simulink model "DiagCCaller_TestHarness"  (R2019a)
settings: Solver=FixedStepDiscrete  StartTime=0.0  StopTime=10.0  FixedStep=0.1  RelTol=1e-3  EnableMultiTasking=on
undefined symbols (not defined in the file): Dem_EventStatusType, sigbuilder_block
(part 1 of 4)
settings Model: Creator=E9911830  LastModifiedBy=E9911830
settings SolverCC: AutoInsertRateTranBlk=on
settings DataIOCC: ReturnWorkspaceOutputs=off
settings OptimizationCC: DefaultParameterBehavior=Inlined  EnhancedBackFolding=on  PassReuseOutputArgsAs=Individual arguments  ZeroExternalMemoryAtStartup=off  ZeroInternalMemoryAtStartup=off  OptimizeBlockOrder=speed  DifferentSizesBufferReuse=on  OptimizationCustomize=off
settings DebuggingCC: ParameterTunabilityLossMsg=error
settings SFSimCC: SimCustomHeaderCode="#include \"DiagDebounce.h\""  SimUserSources=DiagDebounce.c  MATLABDynamicMemAlloc=off
settings RTWCC: SystemTargetFile=ert.tlc  GenCodeOnly=on  TemplateMakefile=ert_default_tmf  GenerateReport=on  IncludeHyperlinkInReport=on  LaunchReport=on  GenerateTraceInfo=on  GenerateTraceReport=on  GenerateTraceReportSl=on  GenerateTraceReportSf=on  GenerateTraceReportEml=on
settings CodeAppCC: ForceParamTrailComments=on  IgnoreCustomStorageClasses=off  OperatorAnnotations=on  SimulinkDataObjDesc=on  SFDataObjDesc=on  InsertBlockDesc=on
settings ERTTargetCC: TargetLangStandard=C99 (ISO)  GenerateSampleERTMain=on  InlinedParameterPlacement=NonHierarchical  ERTCustomFileTemplate=example_file_process.tlc

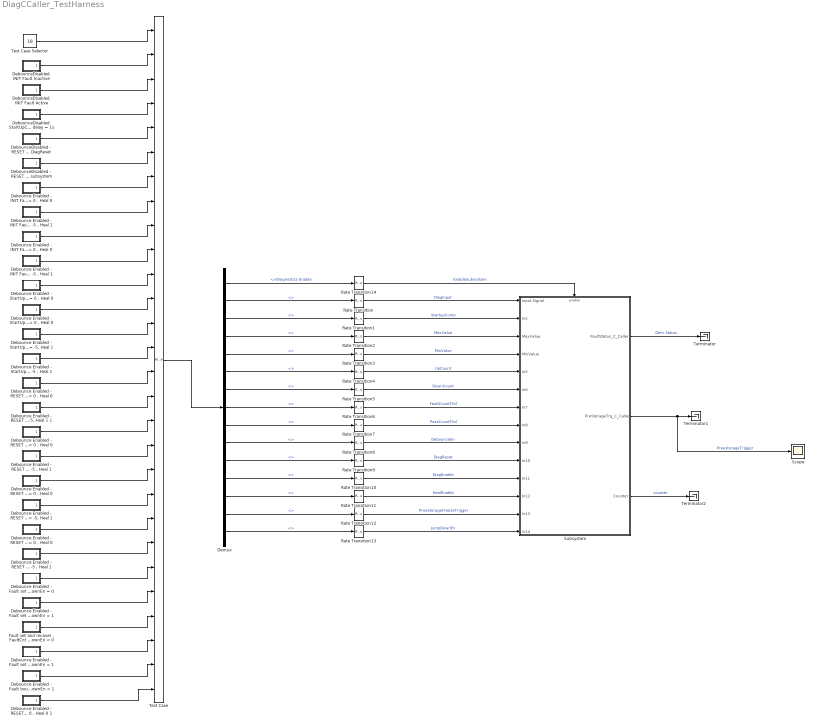
== system DiagCCaller_TestHarness ==
  "Debounce Enabled - Fault bounces , FaultCnt = 10, PassCnt = -5 , Heal =1, JumpDownEn = 1 " : Subsystem
  "Debounce Enabled - Fault set and recover , FaultCnt = 10, PassCnt = -5 , Heal =1, JumpDownEn = 1 " : Subsystem
  "Debounce Enabled - Fault set and recover , FaultCnt = 10, PassCnt = 0 , Heal =0, JumpDownEn = 0 " : Subsystem
  "Debounce Enabled - Fault set and recover , FaultCnt = 10, PassCnt = 0 , Heal =0, JumpDownEn = 1 " : Subsystem
  "Debounce Enabled - INIT Fault Active , FaultCnt = 10, PassCnt = -5 , Heal 1 " : Subsystem
  "Debounce Enabled - INIT Fault Active , FaultCnt = 10, PassCnt = 0 , Heal 0 " : Subsystem
  "Debounce Enabled - INIT Fault Inactive , FaultCnt = 10, PassCnt = -5 , Heal 1 " : Subsystem
  "Debounce Enabled - INIT Fault Inactive , FaultCnt = 10, PassCnt = 0 , Heal 0 " : Subsystem
  "Debounce Enabled - RESET by Calibration ,Fault Active, FaultCnt = 10, PassCnt = -5, Heal 1 1" : Subsystem
  "Debounce Enabled - RESET by Calibration ,Fault Active, FaultCnt = 10, PassCnt = 0 , Heal 0 " : Subsystem
  "Debounce Enabled - RESET by Calibration ,Fault Inactive , FaultCnt = 10, PassCnt = 0 , Heal 0 " : Subsystem
  "Debounce Enabled - RESET by Calibration ,Fault Inactive,  FaultCnt = 10, PassCnt = -5 , Heal 1 " : Subsystem
  "Debounce Enabled - RESET by Disable\\Enable subsystem,Fault Active, FaultCnt = 10, PassCnt = -5, Heal 1 " : Subsystem
  "Debounce Enabled - RESET by Disable\\Enable subsystem,Fault Active, FaultCnt = 10, PassCnt = 0 , Heal 0 " : Subsystem
  "Debounce Enabled - RESET by Disable\\Enable subsystem,Fault Inactive,  FaultCnt = 10, PassCnt = -5 , Heal 1 " : Subsystem
  "Debounce Enabled - RESET by Disable\\Enable subsystem,Fault Inactive, , FaultCnt = 10, PassCnt = 0 , Heal 0 " : Subsystem
  "Debounce Enabled - RESET by Disable\\Enable subsystem,Fault Inactive, , FaultCnt = 10, PassCnt = 0 , Heal 0 1" : Subsystem
  "Debounce Enabled - StartUpComp delay = 1s, Fault Active , FaultCnt = 10, PassCnt = -5 , Heal 1 " : Subsystem
  "Debounce Enabled - StartUpComp delay = 1s, Fault Active , FaultCnt = 10, PassCnt = 0 , Heal 0 " : Subsystem
  "Debounce Enabled - StartUpComp delay = 1s, Fault Inactive , FaultCnt = 10, PassCnt = -5, Heal 1 " : Subsystem
  "Debounce Enabled - StartUpComp delay = 1s, Fault Inactive , FaultCnt = 10, PassCnt = 0 , Heal 0 " : Subsystem
  "DebounceDisabled - RESET by Calibration DiagReset " : Subsystem
  "DebounceDisabled - RESET by Disable\\Enable subsystem " : Subsystem
  "DebounceDisabled INIT Fault Active " : Subsystem
  "DebounceDisabled INIT Fault Inactive " : Subsystem
  "DebounceDisabled StartUpComp delay = 1s " : Subsystem
  Demux : Demux  Outputs=15
  "Fault set and recover , FaultCnt = 10, PassCnt = -5 , Heal =1, JumpDownEn = 0 " : Subsystem
  Rate Transition{,1..14} (15 alike) : RateTransition  OutPortSampleTime=.1
  Scope : Scope
  Subsystem : Subsystem
  Terminator : Terminator
  Terminator1 : Terminator
  Terminator2 : Terminator
  Test Case : MultiPortSwitch  Inputs=27
  Test Case Selector : Constant  Value=18
  wires:
  Rate Transition/1 -> Subsystem/1(Input Signal)  "DiagInput"
  Demux/2 -> Rate Transition/1  "<>"
  Demux/3 -> Rate Transition1/1  "<>"
  Demux/4 -> Rate Transition2/1  "<>"
  Demux/5 -> Rate Transition3/1  "<>"
  Demux/6 -> Rate Transition4/1  "<>"
  Demux/7 -> Rate Transition5/1  "<>"
  Demux/8 -> Rate Transition6/1  "<>"
  Demux/9 -> Rate Transition7/1  "<>"
  Demux/10 -> Rate Transition8/1  "<>"
  Demux/11 -> Rate Transition9/1  "<>"
  Demux/12 -> Rate Transition10/1  "<>"
  Demux/13 -> Rate Transition11/1  "<>"
  Demux/14 -> Rate Transition12/1  "<>"
  Demux/15 -> Rate Transition13/1  "<>"
  Subsystem/1(FaultStatus_C_Caller) -> Terminator/1  "Dem Status"
  Subsystem/2(PreStorageTrg_C_Caller) -> Scope/1, Terminator1/1  "PreestorageTrigger"
  Demux/1 -> Rate Transition14/1  "<>Diagnostics Enable"
  "DebounceDisabled INIT Fault Inactive "/1(Out1) -> Test Case/2
  Test Case/1 -> Demux/1
  Test Case Selector/1 -> Test Case/1
  "DebounceDisabled INIT Fault Active "/1(Out1) -> Test Case/3
  "DebounceDisabled StartUpComp delay = 1s "/1(Out1) -> Test Case/4
  Rate Transition1/1 -> Subsystem/2(In2)  "StartupComp"
  Rate Transition4/1 -> Subsystem/5(In5)  "UpCount"
  Rate Transition5/1 -> Subsystem/6(In6)  "DownCount"
  Rate Transition6/1 -> Subsystem/7(In7)  "FaultCountThd"
  Rate Transition7/1 -> Subsystem/8(In8)  "PassCountThd"
  Rate Transition8/1 -> Subsystem/9(In9)  "DebounceEn"
  Rate Transition9/1 -> Subsystem/10(In10)  "DiagReset"
  Rate Transition10/1 -> Subsystem/11(In11)  "DiagEnable"
  Rate Transition11/1 -> Subsystem/12(In12)  "HealEnable"
  Rate Transition12/1 -> Subsystem/13(In13)  "PreestorageFreezeTrigger"
  Rate Transition13/1 -> Subsystem/14(In14)  "JumpDownEn"
  Rate Transition14/1 -> Subsystem/Enable  "EnableSubsystem"
  "DebounceDisabled - RESET by Calibration DiagReset "/1(Out1) -> Test Case/5
  Subsystem/3(Counter) -> Terminator2/1  "counter"
  "DebounceDisabled - RESET by Disable\\Enable subsystem "/1(Out1) -> Test Case/6
  "Debounce Enabled - INIT Fault Inactive , FaultCnt = 10, PassCnt = 0 , Heal 0 "/1(Out1) -> Test Case/7
  "Debounce Enabled - INIT Fault Inactive , FaultCnt = 10, PassCnt = -5 , Heal 1 "/1(Out1) -> Test Case/8
  "Debounce Enabled - INIT Fault Active , FaultCnt = 10, PassCnt = 0 , Heal 0 "/1(Out1) -> Test Case/9
  "Debounce Enabled - INIT Fault Active , FaultCnt = 10, PassCnt = -5 , Heal 1 "/1(Out1) -> Test Case/10
  "Debounce Enabled - StartUpComp delay = 1s, Fault Inactive , FaultCnt = 10, PassCnt = 0 , Heal 0 "/1(Out1) -> Test Case/11
  "Debounce Enabled - StartUpComp delay = 1s, Fault Active , FaultCnt = 10, PassCnt = 0 , Heal 0 "/1(Out1) -> Test Case/12
  "Debounce Enabled - StartUpComp delay = 1s, Fault Inactive , FaultCnt = 10, PassCnt = -5, Heal 1 "/1(Out1) -> Test Case/13
  "Debounce Enabled - StartUpComp delay = 1s, Fault Active , FaultCnt = 10, PassCnt = -5 , Heal 1 "/1(Out1) -> Test Case/14
  "Debounce Enabled - RESET by Calibration ,Fault Active, FaultCnt = 10, PassCnt = 0 , Heal 0 "/1(Out1) -> Test Case/15
  "Debounce Enabled - RESET by Calibration ,Fault Active, FaultCnt = 10, PassCnt = -5, Heal 1 1"/1(Out1) -> Test Case/16
  "Debounce Enabled - RESET by Calibration ,Fault Inactive , FaultCnt = 10, PassCnt = 0 , Heal 0 "/1(Out1) -> Test Case/17
  "Debounce Enabled - RESET by Calibration ,Fault Inactive,  FaultCnt = 10, PassCnt = -5 , Heal 1 "/1(Out1) -> Test Case/18
  "Debounce Enabled - RESET by Disable\\Enable subsystem,Fault Active, FaultCnt = 10, PassCnt = 0 , Heal 0 "/1(Out1) -> Test Case/19
  "Debounce Enabled - RESET by Disable\\Enable subsystem,Fault Active, FaultCnt = 10, PassCnt = -5, Heal 1 "/1(Out1) -> Test Case/20
  "Debounce Enabled - RESET by Disable\\Enable subsystem,Fault Inactive, , FaultCnt = 10, PassCnt = 0 , Heal 0 "/1(Out1) -> Test Case/21
  "Debounce Enabled - RESET by Disable\\Enable subsystem,Fault Inactive,  FaultCnt = 10, PassCnt = -5 , Heal 1 "/1(Out1) -> Test Case/22
  "Debounce Enabled - Fault set and recover , FaultCnt = 10, PassCnt = 0 , Heal =0, JumpDownEn = 1 "/1(Out1) -> Test Case/24
  "Debounce Enabled - Fault set and recover , FaultCnt = 10, PassCnt = 0 , Heal =0, JumpDownEn = 0 "/1(Out1) -> Test Case/23
  "Fault set and recover , FaultCnt = 10, PassCnt = -5 , Heal =1, JumpDownEn = 0 "/1(Out1) -> Test Case/25
  "Debounce Enabled - Fault set and recover , FaultCnt = 10, PassCnt = -5 , Heal =1, JumpDownEn = 1 "/1(Out1) -> Test Case/26
  "Debounce Enabled - Fault bounces , FaultCnt = 10, PassCnt = -5 , Heal =1, JumpDownEn = 1 "/1(Out1) -> Test Case/27
  Rate Transition2/1 -> Subsystem/3(MaxValue)  "MaxValue"
  Rate Transition3/1 -> Subsystem/4(MinValue)  "MinValue"
  "Debounce Enabled - RESET by Disable\\Enable subsystem,Fault Inactive, , FaultCnt = 10, PassCnt = 0 , Heal 0 1"/1(Out1) -> Test Case/28

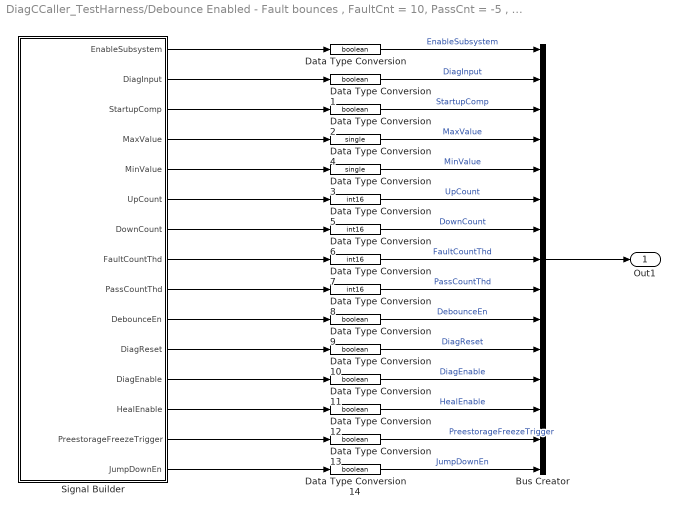
== system DiagCCaller_TestHarness/Debounce Enabled - Fault bounces , FaultCnt = 10, PassCnt = -5 , Heal =1, JumpDownEn = 1  ==
  Bus Creator : BusCreator  Inputs=15
  Data Type Conversion{,1..2,9..14} (9 alike) : DataTypeConversion  OutDataTypeStr=boolean
  Data Type Conversion3 : DataTypeConversion  OutDataTypeStr=single
  Data Type Conversion4 : DataTypeConversion  OutDataTypeStr=single
  Data Type Conversion{5..8} (4 alike) : DataTypeConversion  OutDataTypeStr=int16
  Signal Builder : Subsystem  Tag=STV Subsys  LoadFcn=sigbuilder_block('load');  StartFcn=sigbuilder_block('start');  StopFcn=sigbuilder_block('stop');  ClipboardFcn=sigbuilder_block('clipboard');  TreatAsAtomicUnit=on  mask(Sigbuilder block){tuvar=[0:10]}
      mask help: Simulink:masks:SigbuilderBlock_MD
      mask init:
      | if ~strcmp(get_param(bdroot(gcbh),'SimulationStatus'),'stopped') tuvar = sigbuilder_block('maskInit'); end
      settings: CopyFcn=sigbuilder_block('copy');  DeleteFcn=sigbuilder_block('delete');  ModelCloseFcn=sigbuilder_block('modelClose');  PreSaveFcn=sigbuilder_block('preSave');  PauseFcn=sigbuilder_block('pause');  ContinueFcn=sigbuilder_block('continue');  NameChangeFcn=sigbuilder_block('namechange');  OpenFcn=sigbuilder_block('open',[0 30 1152 561.6 ]);  CloseFcn=sigbuilder_block('close');
      mask Display: plot(0, 0, 100, 100,[2, 2, 32, 32, 2], [68, 8, 8, 68, 68],[32, 2], [38, 38], [32, 19, 2],[53, 60, 44], [32, 17, 17, 2],[16, 16, 31, 31]);txt = getActiveGroup(gcbh);text(2, 100, txt,'verticalAlignment', 'top');
  Out1 : Outport
  wires:
  Bus Creator/1 -> Out1/1
  Signal Builder/2(DiagInput) -> Data Type Conversion1/1
  Signal Builder/3(StartupComp) -> Data Type Conversion2/1
  Signal Builder/4(MaxValue) -> Data Type Conversion4/1
  Signal Builder/5(MinValue) -> Data Type Conversion3/1
  Signal Builder/6(UpCount) -> Data Type Conversion5/1
  Signal Builder/7(DownCount) -> Data Type Conversion6/1
  Signal Builder/8(FaultCountThd) -> Data Type Conversion7/1
  Signal Builder/9(PassCountThd) -> Data Type Conversion8/1
  Signal Builder/10(DebounceEn) -> Data Type Conversion9/1
  Signal Builder/11(DiagReset) -> Data Type Conversion10/1
  Signal Builder/12(DiagEnable) -> Data Type Conversion11/1
  Signal Builder/13(HealEnable) -> Data Type Conversion12/1
  Signal Builder/14(PreestorageFreezeTrigger) -> Data Type Conversion13/1
  Signal Builder/15(JumpDownEn) -> Data Type Conversion14/1
  Signal Builder/1(EnableSubsystem) -> Data Type Conversion/1
  Data Type Conversion/1 -> Bus Creator/1  "EnableSubsystem"
  Data Type Conversion1/1 -> Bus Creator/2  "DiagInput"
  Data Type Conversion2/1 -> Bus Creator/3  "StartupComp"
  Data Type Conversion4/1 -> Bus Creator/4  "MaxValue"
  Data Type Conversion3/1 -> Bus Creator/5  "MinValue"
  Data Type Conversion5/1 -> Bus Creator/6  "UpCount"
  Data Type Conversion6/1 -> Bus Creator/7  "DownCount"
  Data Type Conversion7/1 -> Bus Creator/8  "FaultCountThd"
  Data Type Conversion8/1 -> Bus Creator/9  "PassCountThd"
  Data Type Conversion9/1 -> Bus Creator/10  "DebounceEn"
  Data Type Conversion10/1 -> Bus Creator/11  "DiagReset"
  Data Type Conversion11/1 -> Bus Creator/12  "DiagEnable"
  Data Type Conversion12/1 -> Bus Creator/13  "HealEnable"
  Data Type Conversion13/1 -> Bus Creator/14  "PreestorageFreezeTrigger"
  Data Type Conversion14/1 -> Bus Creator/15  "JumpDownEn"

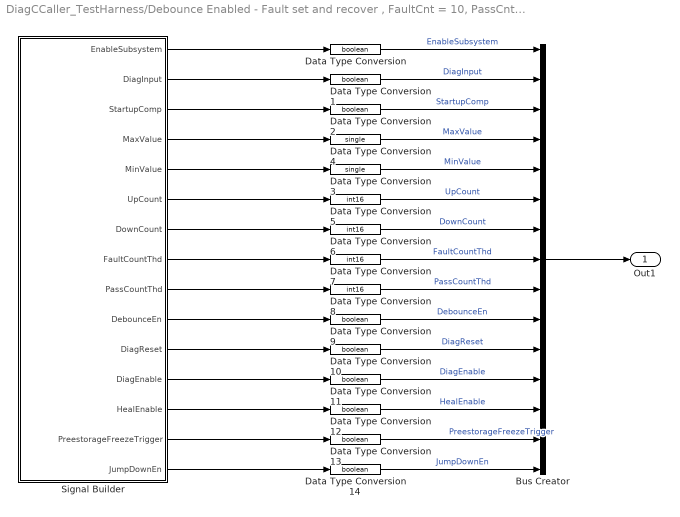
== system DiagCCaller_TestHarness/Debounce Enabled - Fault set and recover , FaultCnt = 10, PassCnt = -5 , Heal =1, JumpDownEn = 1  ==
  Bus Creator : BusCreator  Inputs=15
  Data Type Conversion{,1..2,9..14} (9 alike) : DataTypeConversion  OutDataTypeStr=boolean
  Data Type Conversion3 : DataTypeConversion  OutDataTypeStr=single
  Data Type Conversion4 : DataTypeConversion  OutDataTypeStr=single
  Data Type Conversion{5..8} (4 alike) : DataTypeConversion  OutDataTypeStr=int16
  Signal Builder : Subsystem  Tag=STV Subsys  LoadFcn=sigbuilder_block('load');  StartFcn=sigbuilder_block('start');  StopFcn=sigbuilder_block('stop');  ClipboardFcn=sigbuilder_block('clipboard');  TreatAsAtomicUnit=on  mask(Sigbuilder block){tuvar=[0:10]}
      mask help: Simulink:masks:SigbuilderBlock_MD
      mask init:
      | if ~strcmp(get_param(bdroot(gcbh),'SimulationStatus'),'stopped') tuvar = sigbuilder_block('maskInit'); end
      settings: CopyFcn=sigbuilder_block('copy');  DeleteFcn=sigbuilder_block('delete');  ModelCloseFcn=sigbuilder_block('modelClose');  PreSaveFcn=sigbuilder_block('preSave');  PauseFcn=sigbuilder_block('pause');  ContinueFcn=sigbuilder_block('continue');  NameChangeFcn=sigbuilder_block('namechange');  OpenFcn=sigbuilder_block('open',[5.4 30 1141.2 522.6 ]);  CloseFcn=sigbuilder_block('close');
      mask Display: plot(0, 0, 100, 100,[2, 2, 32, 32, 2], [68, 8, 8, 68, 68],[32, 2], [38, 38], [32, 19, 2],[53, 60, 44], [32, 17, 17, 2],[16, 16, 31, 31]);txt = getActiveGroup(gcbh);text(2, 100, txt,'verticalAlignment', 'top');
  Out1 : Outport
  wires:
  Data Type Conversion14/1 -> Bus Creator/15  "JumpDownEn"
  Data Type Conversion13/1 -> Bus Creator/14  "PreestorageFreezeTrigger"
  Data Type Conversion12/1 -> Bus Creator/13  "HealEnable"
  Data Type Conversion11/1 -> Bus Creator/12  "DiagEnable"
  Data Type Conversion10/1 -> Bus Creator/11  "DiagReset"
  Data Type Conversion9/1 -> Bus Creator/10  "DebounceEn"
  Data Type Conversion8/1 -> Bus Creator/9  "PassCountThd"
  Data Type Conversion7/1 -> Bus Creator/8  "FaultCountThd"
  Data Type Conversion6/1 -> Bus Creator/7  "DownCount"
  Data Type Conversion5/1 -> Bus Creator/6  "UpCount"
  Data Type Conversion3/1 -> Bus Creator/5  "MinValue"
  Data Type Conversion4/1 -> Bus Creator/4  "MaxValue"
  Data Type Conversion2/1 -> Bus Creator/3  "StartupComp"
  Data Type Conversion1/1 -> Bus Creator/2  "DiagInput"
  Data Type Conversion/1 -> Bus Creator/1  "EnableSubsystem"
  Signal Builder/1(EnableSubsystem) -> Data Type Conversion/1
  Signal Builder/15(JumpDownEn) -> Data Type Conversion14/1
  Signal Builder/14(PreestorageFreezeTrigger) -> Data Type Conversion13/1
  Signal Builder/13(HealEnable) -> Data Type Conversion12/1
  Signal Builder/12(DiagEnable) -> Data Type Conversion11/1
  Signal Builder/11(DiagReset) -> Data Type Conversion10/1
  Signal Builder/10(DebounceEn) -> Data Type Conversion9/1
  Signal Builder/9(PassCountThd) -> Data Type Conversion8/1
  Signal Builder/8(FaultCountThd) -> Data Type Conversion7/1
  Signal Builder/7(DownCount) -> Data Type Conversion6/1
  Signal Builder/6(UpCount) -> Data Type Conversion5/1
  Signal Builder/5(MinValue) -> Data Type Conversion3/1
  Signal Builder/4(MaxValue) -> Data Type Conversion4/1
  Signal Builder/3(StartupComp) -> Data Type Conversion2/1
  Signal Builder/2(DiagInput) -> Data Type Conversion1/1
  Bus Creator/1 -> Out1/1

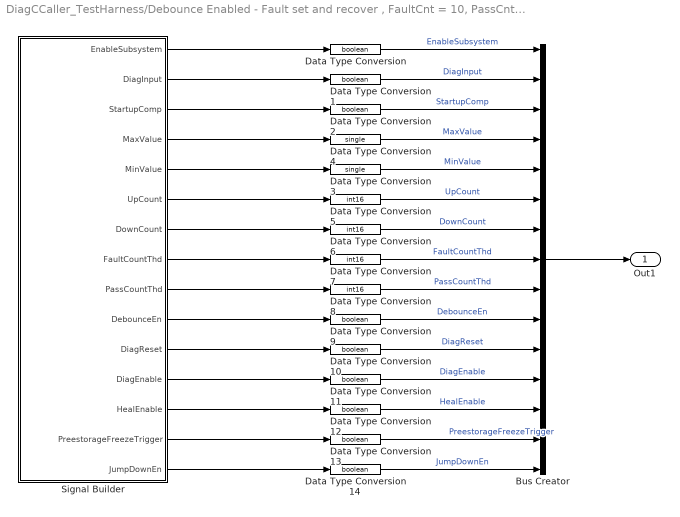
== system DiagCCaller_TestHarness/Debounce Enabled - Fault set and recover , FaultCnt = 10, PassCnt = 0 , Heal =0, JumpDownEn = 0  ==
  Bus Creator : BusCreator  Inputs=15
  Data Type Conversion{,1..2,9..14} (9 alike) : DataTypeConversion  OutDataTypeStr=boolean
  Data Type Conversion3 : DataTypeConversion  OutDataTypeStr=single
  Data Type Conversion4 : DataTypeConversion  OutDataTypeStr=single
  Data Type Conversion{5..8} (4 alike) : DataTypeConversion  OutDataTypeStr=int16
  Signal Builder : Subsystem  Tag=STV Subsys  LoadFcn=sigbuilder_block('load');  StartFcn=sigbuilder_block('start');  StopFcn=sigbuilder_block('stop');  ClipboardFcn=sigbuilder_block('clipboard');  TreatAsAtomicUnit=on  mask(Sigbuilder block){tuvar=[0:10]}
      mask help: Simulink:masks:SigbuilderBlock_MD
      mask init:
      | if ~strcmp(get_param(bdroot(gcbh),'SimulationStatus'),'stopped') tuvar = sigbuilder_block('maskInit'); end
      settings: CopyFcn=sigbuilder_block('copy');  DeleteFcn=sigbuilder_block('delete');  ModelCloseFcn=sigbuilder_block('modelClose');  PreSaveFcn=sigbuilder_block('preSave');  PauseFcn=sigbuilder_block('pause');  ContinueFcn=sigbuilder_block('continue');  NameChangeFcn=sigbuilder_block('namechange');  OpenFcn=sigbuilder_block('open',[5.4 30 1141.2 522.6 ]);  CloseFcn=sigbuilder_block('close');
      mask Display: plot(0, 0, 100, 100,[2, 2, 32, 32, 2], [68, 8, 8, 68, 68],[32, 2], [38, 38], [32, 19, 2],[53, 60, 44], [32, 17, 17, 2],[16, 16, 31, 31]);txt = getActiveGroup(gcbh);text(2, 100, txt,'verticalAlignment', 'top');
  Out1 : Outport
  wires:
  Data Type Conversion14/1 -> Bus Creator/15  "JumpDownEn"
  Data Type Conversion13/1 -> Bus Creator/14  "PreestorageFreezeTrigger"
  Data Type Conversion12/1 -> Bus Creator/13  "HealEnable"
  Data Type Conversion11/1 -> Bus Creator/12  "DiagEnable"
  Data Type Conversion10/1 -> Bus Creator/11  "DiagReset"
  Data Type Conversion9/1 -> Bus Creator/10  "DebounceEn"
  Data Type Conversion8/1 -> Bus Creator/9  "PassCountThd"
  Data Type Conversion7/1 -> Bus Creator/8  "FaultCountThd"
  Data Type Conversion6/1 -> Bus Creator/7  "DownCount"
  Data Type Conversion5/1 -> Bus Creator/6  "UpCount"
  Data Type Conversion3/1 -> Bus Creator/5  "MinValue"
  Data Type Conversion4/1 -> Bus Creator/4  "MaxValue"
  Data Type Conversion2/1 -> Bus Creator/3  "StartupComp"
  Data Type Conversion1/1 -> Bus Creator/2  "DiagInput"
  Data Type Conversion/1 -> Bus Creator/1  "EnableSubsystem"
  Signal Builder/1(EnableSubsystem) -> Data Type Conversion/1
  Signal Builder/15(JumpDownEn) -> Data Type Conversion14/1
  Signal Builder/14(PreestorageFreezeTrigger) -> Data Type Conversion13/1
  Signal Builder/13(HealEnable) -> Data Type Conversion12/1
  Signal Builder/12(DiagEnable) -> Data Type Conversion11/1
  Signal Builder/11(DiagReset) -> Data Type Conversion10/1
  Signal Builder/10(DebounceEn) -> Data Type Conversion9/1
  Signal Builder/9(PassCountThd) -> Data Type Conversion8/1
  Signal Builder/8(FaultCountThd) -> Data Type Conversion7/1
  Signal Builder/7(DownCount) -> Data Type Conversion6/1
  Signal Builder/6(UpCount) -> Data Type Conversion5/1
  Signal Builder/5(MinValue) -> Data Type Conversion3/1
  Signal Builder/4(MaxValue) -> Data Type Conversion4/1
  Signal Builder/3(StartupComp) -> Data Type Conversion2/1
  Signal Builder/2(DiagInput) -> Data Type Conversion1/1
  Bus Creator/1 -> Out1/1

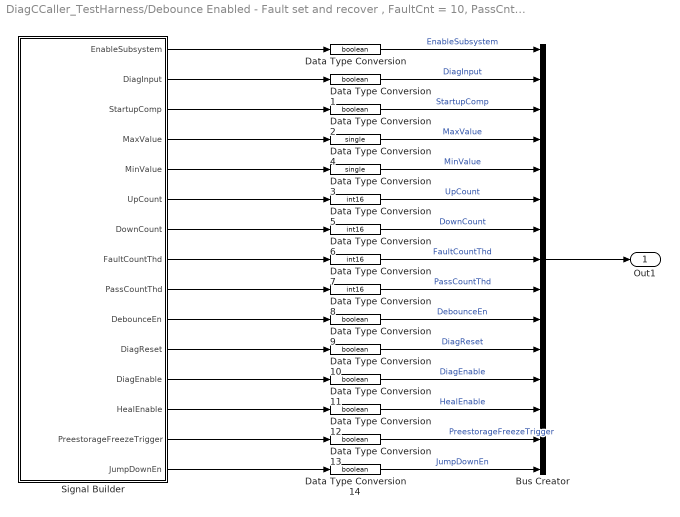
== system DiagCCaller_TestHarness/Debounce Enabled - Fault set and recover , FaultCnt = 10, PassCnt = 0 , Heal =0, JumpDownEn = 1  ==
  Bus Creator : BusCreator  Inputs=15
  Data Type Conversion{,1..2,9..14} (9 alike) : DataTypeConversion  OutDataTypeStr=boolean
  Data Type Conversion3 : DataTypeConversion  OutDataTypeStr=single
  Data Type Conversion4 : DataTypeConversion  OutDataTypeStr=single
  Data Type Conversion{5..8} (4 alike) : DataTypeConversion  OutDataTypeStr=int16
  Signal Builder : Subsystem  Tag=STV Subsys  LoadFcn=sigbuilder_block('load');  StartFcn=sigbuilder_block('start');  StopFcn=sigbuilder_block('stop');  ClipboardFcn=sigbuilder_block('clipboard');  TreatAsAtomicUnit=on  mask(Sigbuilder block){tuvar=[0:10]}
      mask help: Simulink:masks:SigbuilderBlock_MD
      mask init:
      | if ~strcmp(get_param(bdroot(gcbh),'SimulationStatus'),'stopped') tuvar = sigbuilder_block('maskInit'); end
      settings: CopyFcn=sigbuilder_block('copy');  DeleteFcn=sigbuilder_block('delete');  ModelCloseFcn=sigbuilder_block('modelClose');  PreSaveFcn=sigbuilder_block('preSave');  PauseFcn=sigbuilder_block('pause');  ContinueFcn=sigbuilder_block('continue');  NameChangeFcn=sigbuilder_block('namechange');  OpenFcn=sigbuilder_block('open',[5.4 30 1141.2 522.6 ]);  CloseFcn=sigbuilder_block('close');
      mask Display: plot(0, 0, 100, 100,[2, 2, 32, 32, 2], [68, 8, 8, 68, 68],[32, 2], [38, 38], [32, 19, 2],[53, 60, 44], [32, 17, 17, 2],[16, 16, 31, 31]);txt = getActiveGroup(gcbh);text(2, 100, txt,'verticalAlignment', 'top');
  Out1 : Outport
  wires:
  Bus Creator/1 -> Out1/1
  Signal Builder/2(DiagInput) -> Data Type Conversion1/1
  Signal Builder/3(StartupComp) -> Data Type Conversion2/1
  Signal Builder/4(MaxValue) -> Data Type Conversion4/1
  Signal Builder/5(MinValue) -> Data Type Conversion3/1
  Signal Builder/6(UpCount) -> Data Type Conversion5/1
  Signal Builder/7(DownCount) -> Data Type Conversion6/1
  Signal Builder/8(FaultCountThd) -> Data Type Conversion7/1
  Signal Builder/9(PassCountThd) -> Data Type Conversion8/1
  Signal Builder/10(DebounceEn) -> Data Type Conversion9/1
  Signal Builder/11(DiagReset) -> Data Type Conversion10/1
  Signal Builder/12(DiagEnable) -> Data Type Conversion11/1
  Signal Builder/13(HealEnable) -> Data Type Conversion12/1
  Signal Builder/14(PreestorageFreezeTrigger) -> Data Type Conversion13/1
  Signal Builder/15(JumpDownEn) -> Data Type Conversion14/1
  Signal Builder/1(EnableSubsystem) -> Data Type Conversion/1
  Data Type Conversion/1 -> Bus Creator/1  "EnableSubsystem"
  Data Type Conversion1/1 -> Bus Creator/2  "DiagInput"
  Data Type Conversion2/1 -> Bus Creator/3  "StartupComp"
  Data Type Conversion4/1 -> Bus Creator/4  "MaxValue"
  Data Type Conversion3/1 -> Bus Creator/5  "MinValue"
  Data Type Conversion5/1 -> Bus Creator/6  "UpCount"
  Data Type Conversion6/1 -> Bus Creator/7  "DownCount"
  Data Type Conversion7/1 -> Bus Creator/8  "FaultCountThd"
  Data Type Conversion8/1 -> Bus Creator/9  "PassCountThd"
  Data Type Conversion9/1 -> Bus Creator/10  "DebounceEn"
  Data Type Conversion10/1 -> Bus Creator/11  "DiagReset"
  Data Type Conversion11/1 -> Bus Creator/12  "DiagEnable"
  Data Type Conversion12/1 -> Bus Creator/13  "HealEnable"
  Data Type Conversion13/1 -> Bus Creator/14  "PreestorageFreezeTrigger"
  Data Type Conversion14/1 -> Bus Creator/15  "JumpDownEn"

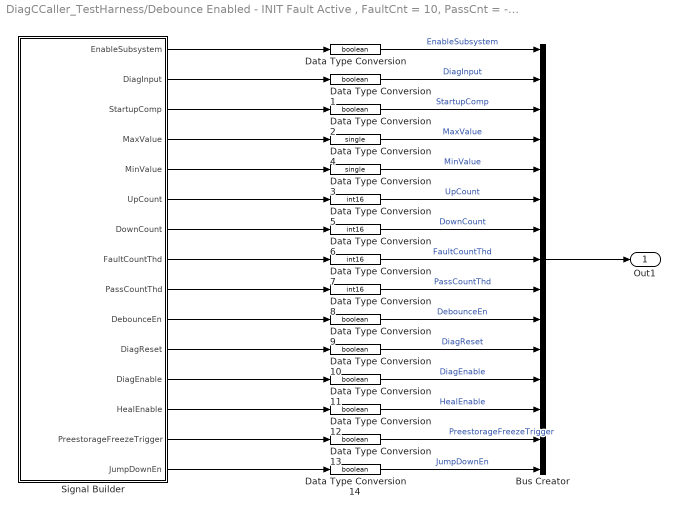
== system DiagCCaller_TestHarness/Debounce Enabled - INIT Fault Active , FaultCnt = 10, PassCnt = -5 , Heal 1  ==
  Bus Creator : BusCreator  Inputs=15
  Data Type Conversion{,1..2,9..14} (9 alike) : DataTypeConversion  OutDataTypeStr=boolean
  Data Type Conversion3 : DataTypeConversion  OutDataTypeStr=single
  Data Type Conversion4 : DataTypeConversion  OutDataTypeStr=single
  Data Type Conversion{5..8} (4 alike) : DataTypeConversion  OutDataTypeStr=int16
  Signal Builder : Subsystem  Tag=STV Subsys  LoadFcn=sigbuilder_block('load');  StartFcn=sigbuilder_block('start');  StopFcn=sigbuilder_block('stop');  ClipboardFcn=sigbuilder_block('clipboard');  TreatAsAtomicUnit=on  mask(Sigbuilder block){tuvar=[0:10]}
      mask help: Simulink:masks:SigbuilderBlock_MD
      mask init:
      | if ~strcmp(get_param(bdroot(gcbh),'SimulationStatus'),'stopped') tuvar = sigbuilder_block('maskInit'); end
      settings: CopyFcn=sigbuilder_block('copy');  DeleteFcn=sigbuilder_block('delete');  ModelCloseFcn=sigbuilder_block('modelClose');  PreSaveFcn=sigbuilder_block('preSave');  PauseFcn=sigbuilder_block('pause');  ContinueFcn=sigbuilder_block('continue');  NameChangeFcn=sigbuilder_block('namechange');  OpenFcn=sigbuilder_block('open',[0 30 1152 561.6 ]);  CloseFcn=sigbuilder_block('close');
      mask Display: plot(0, 0, 100, 100,[2, 2, 32, 32, 2], [68, 8, 8, 68, 68],[32, 2], [38, 38], [32, 19, 2],[53, 60, 44], [32, 17, 17, 2],[16, 16, 31, 31]);txt = getActiveGroup(gcbh);text(2, 100, txt,'verticalAlignment', 'top');
  Out1 : Outport
  wires:
  Data Type Conversion14/1 -> Bus Creator/15  "JumpDownEn"
  Data Type Conversion13/1 -> Bus Creator/14  "PreestorageFreezeTrigger"
  Data Type Conversion12/1 -> Bus Creator/13  "HealEnable"
  Data Type Conversion11/1 -> Bus Creator/12  "DiagEnable"
  Data Type Conversion10/1 -> Bus Creator/11  "DiagReset"
  Data Type Conversion9/1 -> Bus Creator/10  "DebounceEn"
  Data Type Conversion8/1 -> Bus Creator/9  "PassCountThd"
  Data Type Conversion7/1 -> Bus Creator/8  "FaultCountThd"
  Data Type Conversion6/1 -> Bus Creator/7  "DownCount"
  Data Type Conversion5/1 -> Bus Creator/6  "UpCount"
  Data Type Conversion3/1 -> Bus Creator/5  "MinValue"
  Data Type Conversion4/1 -> Bus Creator/4  "MaxValue"
  Data Type Conversion2/1 -> Bus Creator/3  "StartupComp"
  Data Type Conversion1/1 -> Bus Creator/2  "DiagInput"
  Data Type Conversion/1 -> Bus Creator/1  "EnableSubsystem"
  Signal Builder/1(EnableSubsystem) -> Data Type Conversion/1
  Signal Builder/15(JumpDownEn) -> Data Type Conversion14/1
  Signal Builder/14(PreestorageFreezeTrigger) -> Data Type Conversion13/1
  Signal Builder/13(HealEnable) -> Data Type Conversion12/1
  Signal Builder/12(DiagEnable) -> Data Type Conversion11/1
  Signal Builder/11(DiagReset) -> Data Type Conversion10/1
  Signal Builder/10(DebounceEn) -> Data Type Conversion9/1
  Signal Builder/9(PassCountThd) -> Data Type Conversion8/1
  Signal Builder/8(FaultCountThd) -> Data Type Conversion7/1
  Signal Builder/7(DownCount) -> Data Type Conversion6/1
  Signal Builder/6(UpCount) -> Data Type Conversion5/1
  Signal Builder/5(MinValue) -> Data Type Conversion3/1
  Signal Builder/4(MaxValue) -> Data Type Conversion4/1
  Signal Builder/3(StartupComp) -> Data Type Conversion2/1
  Signal Builder/2(DiagInput) -> Data Type Conversion1/1
  Bus Creator/1 -> Out1/1

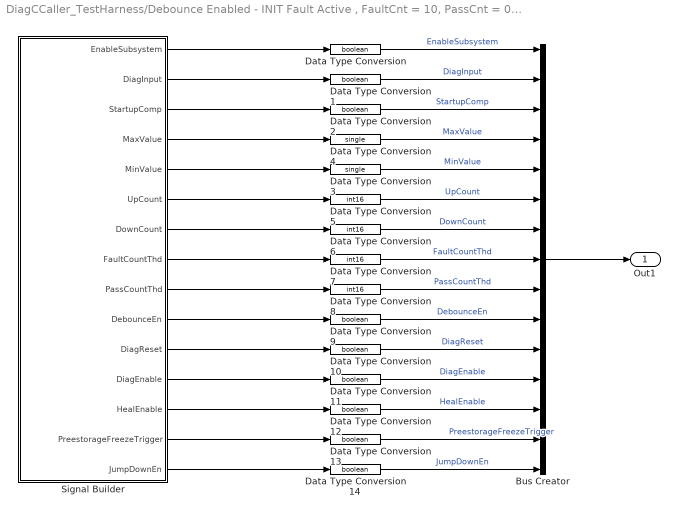
== system DiagCCaller_TestHarness/Debounce Enabled - INIT Fault Active , FaultCnt = 10, PassCnt = 0 , Heal 0  ==
  Bus Creator : BusCreator  Inputs=15
  Data Type Conversion{,1..2,9..14} (9 alike) : DataTypeConversion  OutDataTypeStr=boolean
  Data Type Conversion3 : DataTypeConversion  OutDataTypeStr=single
  Data Type Conversion4 : DataTypeConversion  OutDataTypeStr=single
  Data Type Conversion{5..8} (4 alike) : DataTypeConversion  OutDataTypeStr=int16
  Signal Builder : Subsystem  Tag=STV Subsys  LoadFcn=sigbuilder_block('load');  StartFcn=sigbuilder_block('start');  StopFcn=sigbuilder_block('stop');  ClipboardFcn=sigbuilder_block('clipboard');  TreatAsAtomicUnit=on  mask(Sigbuilder block){tuvar=[0:10]}
      mask help: Simulink:masks:SigbuilderBlock_MD
      mask init:
      | if ~strcmp(get_param(bdroot(gcbh),'SimulationStatus'),'stopped') tuvar = sigbuilder_block('maskInit'); end
      settings: CopyFcn=sigbuilder_block('copy');  DeleteFcn=sigbuilder_block('delete');  ModelCloseFcn=sigbuilder_block('modelClose');  PreSaveFcn=sigbuilder_block('preSave');  PauseFcn=sigbuilder_block('pause');  ContinueFcn=sigbuilder_block('continue');  NameChangeFcn=sigbuilder_block('namechange');  OpenFcn=sigbuilder_block('open',[5.4 30 1141.2 522.6 ]);  CloseFcn=sigbuilder_block('close');
      mask Display: plot(0, 0, 100, 100,[2, 2, 32, 32, 2], [68, 8, 8, 68, 68],[32, 2], [38, 38], [32, 19, 2],[53, 60, 44], [32, 17, 17, 2],[16, 16, 31, 31]);txt = getActiveGroup(gcbh);text(2, 100, txt,'verticalAlignment', 'top');
  Out1 : Outport
  wires:
  Data Type Conversion14/1 -> Bus Creator/15  "JumpDownEn"
  Data Type Conversion13/1 -> Bus Creator/14  "PreestorageFreezeTrigger"
  Data Type Conversion12/1 -> Bus Creator/13  "HealEnable"
  Data Type Conversion11/1 -> Bus Creator/12  "DiagEnable"
  Data Type Conversion10/1 -> Bus Creator/11  "DiagReset"
  Data Type Conversion9/1 -> Bus Creator/10  "DebounceEn"
  Data Type Conversion8/1 -> Bus Creator/9  "PassCountThd"
  Data Type Conversion7/1 -> Bus Creator/8  "FaultCountThd"
  Data Type Conversion6/1 -> Bus Creator/7  "DownCount"
  Data Type Conversion5/1 -> Bus Creator/6  "UpCount"
  Data Type Conversion3/1 -> Bus Creator/5  "MinValue"
  Data Type Conversion4/1 -> Bus Creator/4  "MaxValue"
  Data Type Conversion2/1 -> Bus Creator/3  "StartupComp"
  Data Type Conversion1/1 -> Bus Creator/2  "DiagInput"
  Data Type Conversion/1 -> Bus Creator/1  "EnableSubsystem"
  Signal Builder/1(EnableSubsystem) -> Data Type Conversion/1
  Signal Builder/15(JumpDownEn) -> Data Type Conversion14/1
  Signal Builder/14(PreestorageFreezeTrigger) -> Data Type Conversion13/1
  Signal Builder/13(HealEnable) -> Data Type Conversion12/1
  Signal Builder/12(DiagEnable) -> Data Type Conversion11/1
  Signal Builder/11(DiagReset) -> Data Type Conversion10/1
  Signal Builder/10(DebounceEn) -> Data Type Conversion9/1
  Signal Builder/9(PassCountThd) -> Data Type Conversion8/1
  Signal Builder/8(FaultCountThd) -> Data Type Conversion7/1
  Signal Builder/7(DownCount) -> Data Type Conversion6/1
  Signal Builder/6(UpCount) -> Data Type Conversion5/1
  Signal Builder/5(MinValue) -> Data Type Conversion3/1
  Signal Builder/4(MaxValue) -> Data Type Conversion4/1
  Signal Builder/3(StartupComp) -> Data Type Conversion2/1
  Signal Builder/2(DiagInput) -> Data Type Conversion1/1
  Bus Creator/1 -> Out1/1

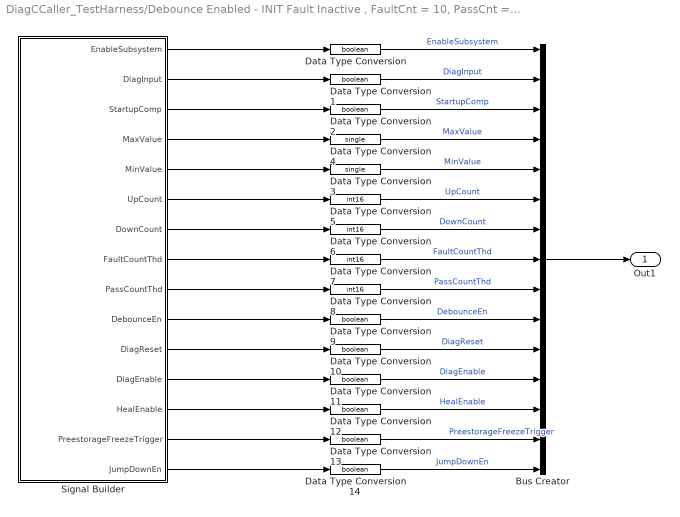
== system DiagCCaller_TestHarness/Debounce Enabled - INIT Fault Inactive , FaultCnt = 10, PassCnt = -5 , Heal 1  ==
  Bus Creator : BusCreator  Inputs=15
  Data Type Conversion{,1..2,9..14} (9 alike) : DataTypeConversion  OutDataTypeStr=boolean
  Data Type Conversion3 : DataTypeConversion  OutDataTypeStr=single
  Data Type Conversion4 : DataTypeConversion  OutDataTypeStr=single
  Data Type Conversion{5..8} (4 alike) : DataTypeConversion  OutDataTypeStr=int16
  Signal Builder : Subsystem  Tag=STV Subsys  LoadFcn=sigbuilder_block('load');  StartFcn=sigbuilder_block('start');  StopFcn=sigbuilder_block('stop');  ClipboardFcn=sigbuilder_block('clipboard');  TreatAsAtomicUnit=on  mask(Sigbuilder block){tuvar=[0:10]}
      mask help: Simulink:masks:SigbuilderBlock_MD
      mask init:
      | if ~strcmp(get_param(bdroot(gcbh),'SimulationStatus'),'stopped') tuvar = sigbuilder_block('maskInit'); end
      settings: CopyFcn=sigbuilder_block('copy');  DeleteFcn=sigbuilder_block('delete');  ModelCloseFcn=sigbuilder_block('modelClose');  PreSaveFcn=sigbuilder_block('preSave');  PauseFcn=sigbuilder_block('pause');  ContinueFcn=sigbuilder_block('continue');  NameChangeFcn=sigbuilder_block('namechange');  OpenFcn=sigbuilder_block('open',[5.4 30 1141.2 522.6 ]);  CloseFcn=sigbuilder_block('close');
      mask Display: plot(0, 0, 100, 100,[2, 2, 32, 32, 2], [68, 8, 8, 68, 68],[32, 2], [38, 38], [32, 19, 2],[53, 60, 44], [32, 17, 17, 2],[16, 16, 31, 31]);txt = getActiveGroup(gcbh);text(2, 100, txt,'verticalAlignment', 'top');
  Out1 : Outport
  wires:
  Bus Creator/1 -> Out1/1
  Signal Builder/2(DiagInput) -> Data Type Conversion1/1
  Signal Builder/3(StartupComp) -> Data Type Conversion2/1
  Signal Builder/4(MaxValue) -> Data Type Conversion4/1
  Signal Builder/5(MinValue) -> Data Type Conversion3/1
  Signal Builder/6(UpCount) -> Data Type Conversion5/1
  Signal Builder/7(DownCount) -> Data Type Conversion6/1
  Signal Builder/8(FaultCountThd) -> Data Type Conversion7/1
  Signal Builder/9(PassCountThd) -> Data Type Conversion8/1
  Signal Builder/10(DebounceEn) -> Data Type Conversion9/1
  Signal Builder/11(DiagReset) -> Data Type Conversion10/1
  Signal Builder/12(DiagEnable) -> Data Type Conversion11/1
  Signal Builder/13(HealEnable) -> Data Type Conversion12/1
  Signal Builder/14(PreestorageFreezeTrigger) -> Data Type Conversion13/1
  Signal Builder/15(JumpDownEn) -> Data Type Conversion14/1
  Signal Builder/1(EnableSubsystem) -> Data Type Conversion/1
  Data Type Conversion/1 -> Bus Creator/1  "EnableSubsystem"
  Data Type Conversion1/1 -> Bus Creator/2  "DiagInput"
  Data Type Conversion2/1 -> Bus Creator/3  "StartupComp"
  Data Type Conversion4/1 -> Bus Creator/4  "MaxValue"
  Data Type Conversion3/1 -> Bus Creator/5  "MinValue"
  Data Type Conversion5/1 -> Bus Creator/6  "UpCount"
  Data Type Conversion6/1 -> Bus Creator/7  "DownCount"
  Data Type Conversion7/1 -> Bus Creator/8  "FaultCountThd"
  Data Type Conversion8/1 -> Bus Creator/9  "PassCountThd"
  Data Type Conversion9/1 -> Bus Creator/10  "DebounceEn"
  Data Type Conversion10/1 -> Bus Creator/11  "DiagReset"
  Data Type Conversion11/1 -> Bus Creator/12  "DiagEnable"
  Data Type Conversion12/1 -> Bus Creator/13  "HealEnable"
  Data Type Conversion13/1 -> Bus Creator/14  "PreestorageFreezeTrigger"
  Data Type Conversion14/1 -> Bus Creator/15  "JumpDownEn"

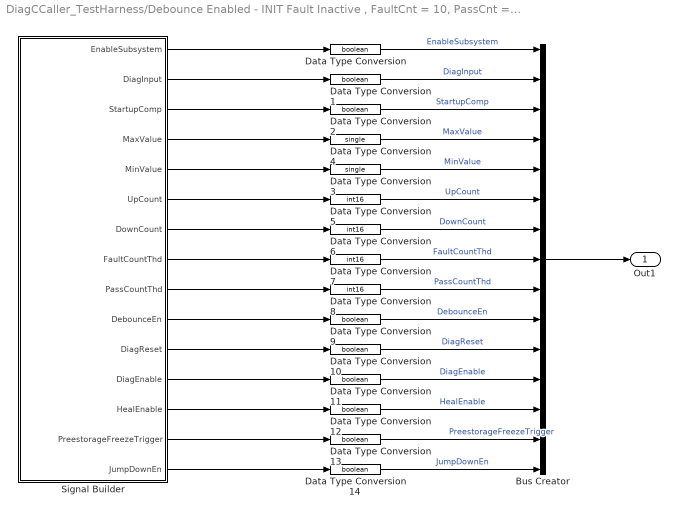
== system DiagCCaller_TestHarness/Debounce Enabled - INIT Fault Inactive , FaultCnt = 10, PassCnt = 0 , Heal 0  ==
  Bus Creator : BusCreator  Inputs=15
  Data Type Conversion{,1..2,9..14} (9 alike) : DataTypeConversion  OutDataTypeStr=boolean
  Data Type Conversion3 : DataTypeConversion  OutDataTypeStr=single
  Data Type Conversion4 : DataTypeConversion  OutDataTypeStr=single
  Data Type Conversion{5..8} (4 alike) : DataTypeConversion  OutDataTypeStr=int16
  Signal Builder : Subsystem  Tag=STV Subsys  LoadFcn=sigbuilder_block('load');  StartFcn=sigbuilder_block('start');  StopFcn=sigbuilder_block('stop');  ClipboardFcn=sigbuilder_block('clipboard');  TreatAsAtomicUnit=on  mask(Sigbuilder block){tuvar=[0:10]}
      mask help: Simulink:masks:SigbuilderBlock_MD
      mask init:
      | if ~strcmp(get_param(bdroot(gcbh),'SimulationStatus'),'stopped') tuvar = sigbuilder_block('maskInit'); end
      settings: CopyFcn=sigbuilder_block('copy');  DeleteFcn=sigbuilder_block('delete');  ModelCloseFcn=sigbuilder_block('modelClose');  PreSaveFcn=sigbuilder_block('preSave');  PauseFcn=sigbuilder_block('pause');  ContinueFcn=sigbuilder_block('continue');  NameChangeFcn=sigbuilder_block('namechange');  OpenFcn=sigbuilder_block('open',[0 30 1152 561.6 ]);  CloseFcn=sigbuilder_block('close');
      mask Display: plot(0, 0, 100, 100,[2, 2, 32, 32, 2], [68, 8, 8, 68, 68],[32, 2], [38, 38], [32, 19, 2],[53, 60, 44], [32, 17, 17, 2],[16, 16, 31, 31]);txt = getActiveGroup(gcbh);text(2, 100, txt,'verticalAlignment', 'top');
  Out1 : Outport
  wires:
  Data Type Conversion14/1 -> Bus Creator/15  "JumpDownEn"
  Data Type Conversion13/1 -> Bus Creator/14  "PreestorageFreezeTrigger"
  Data Type Conversion12/1 -> Bus Creator/13  "HealEnable"
  Data Type Conversion11/1 -> Bus Creator/12  "DiagEnable"
  Data Type Conversion10/1 -> Bus Creator/11  "DiagReset"
  Data Type Conversion9/1 -> Bus Creator/10  "DebounceEn"
  Data Type Conversion8/1 -> Bus Creator/9  "PassCountThd"
  Data Type Conversion7/1 -> Bus Creator/8  "FaultCountThd"
  Data Type Conversion6/1 -> Bus Creator/7  "DownCount"
  Data Type Conversion5/1 -> Bus Creator/6  "UpCount"
  Data Type Conversion3/1 -> Bus Creator/5  "MinValue"
  Data Type Conversion4/1 -> Bus Creator/4  "MaxValue"
  Data Type Conversion2/1 -> Bus Creator/3  "StartupComp"
  Data Type Conversion1/1 -> Bus Creator/2  "DiagInput"
  Data Type Conversion/1 -> Bus Creator/1  "EnableSubsystem"
  Signal Builder/1(EnableSubsystem) -> Data Type Conversion/1
  Signal Builder/15(JumpDownEn) -> Data Type Conversion14/1
  Signal Builder/14(PreestorageFreezeTrigger) -> Data Type Conversion13/1
  Signal Builder/13(HealEnable) -> Data Type Conversion12/1
  Signal Builder/12(DiagEnable) -> Data Type Conversion11/1
  Signal Builder/11(DiagReset) -> Data Type Conversion10/1
  Signal Builder/10(DebounceEn) -> Data Type Conversion9/1
  Signal Builder/9(PassCountThd) -> Data Type Conversion8/1
  Signal Builder/8(FaultCountThd) -> Data Type Conversion7/1
  Signal Builder/7(DownCount) -> Data Type Conversion6/1
  Signal Builder/6(UpCount) -> Data Type Conversion5/1
  Signal Builder/5(MinValue) -> Data Type Conversion3/1
  Signal Builder/4(MaxValue) -> Data Type Conversion4/1
  Signal Builder/3(StartupComp) -> Data Type Conversion2/1
  Signal Builder/2(DiagInput) -> Data Type Conversion1/1
  Bus Creator/1 -> Out1/1

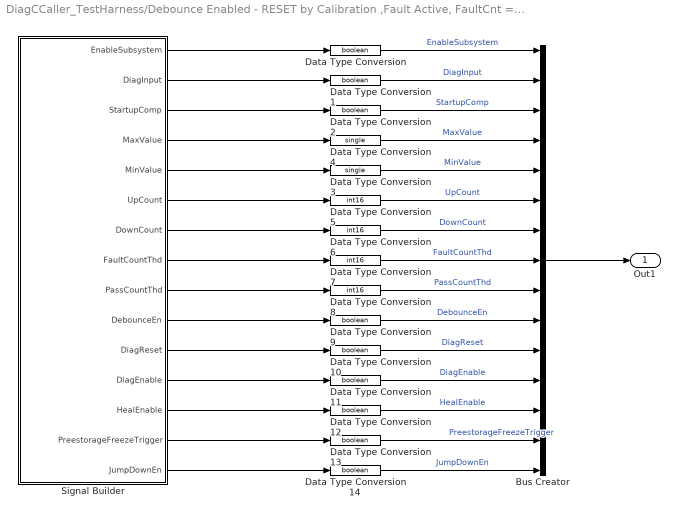
== system DiagCCaller_TestHarness/Debounce Enabled - RESET by Calibration ,Fault Active, FaultCnt = 10, PassCnt = -5, Heal 1 1 ==
  Bus Creator : BusCreator  Inputs=15
  Data Type Conversion{,1..2,9..14} (9 alike) : DataTypeConversion  OutDataTypeStr=boolean
  Data Type Conversion3 : DataTypeConversion  OutDataTypeStr=single
  Data Type Conversion4 : DataTypeConversion  OutDataTypeStr=single
  Data Type Conversion{5..8} (4 alike) : DataTypeConversion  OutDataTypeStr=int16
  Signal Builder : Subsystem  Tag=STV Subsys  LoadFcn=sigbuilder_block('load');  StartFcn=sigbuilder_block('start');  StopFcn=sigbuilder_block('stop');  ClipboardFcn=sigbuilder_block('clipboard');  TreatAsAtomicUnit=on  mask(Sigbuilder block){tuvar=[0:10]}
      mask help: Simulink:masks:SigbuilderBlock_MD
      mask init:
      | if ~strcmp(get_param(bdroot(gcbh),'SimulationStatus'),'stopped') tuvar = sigbuilder_block('maskInit'); end
      settings: CopyFcn=sigbuilder_block('copy');  DeleteFcn=sigbuilder_block('delete');  ModelCloseFcn=sigbuilder_block('modelClose');  PreSaveFcn=sigbuilder_block('preSave');  PauseFcn=sigbuilder_block('pause');  ContinueFcn=sigbuilder_block('continue');  NameChangeFcn=sigbuilder_block('namechange');  OpenFcn=sigbuilder_block('open',[5.4 30 1141.2 522.6 ]);  CloseFcn=sigbuilder_block('close');
      mask Display: plot(0, 0, 100, 100,[2, 2, 32, 32, 2], [68, 8, 8, 68, 68],[32, 2], [38, 38], [32, 19, 2],[53, 60, 44], [32, 17, 17, 2],[16, 16, 31, 31]);txt = getActiveGroup(gcbh);text(2, 100, txt,'verticalAlignment', 'top');
  Out1 : Outport
  wires:
  Data Type Conversion14/1 -> Bus Creator/15  "JumpDownEn"
  Data Type Conversion13/1 -> Bus Creator/14  "PreestorageFreezeTrigger"
  Data Type Conversion12/1 -> Bus Creator/13  "HealEnable"
  Data Type Conversion11/1 -> Bus Creator/12  "DiagEnable"
  Data Type Conversion10/1 -> Bus Creator/11  "DiagReset"
  Data Type Conversion9/1 -> Bus Creator/10  "DebounceEn"
  Data Type Conversion8/1 -> Bus Creator/9  "PassCountThd"
  Data Type Conversion7/1 -> Bus Creator/8  "FaultCountThd"
  Data Type Conversion6/1 -> Bus Creator/7  "DownCount"
  Data Type Conversion5/1 -> Bus Creator/6  "UpCount"
  Data Type Conversion3/1 -> Bus Creator/5  "MinValue"
  Data Type Conversion4/1 -> Bus Creator/4  "MaxValue"
  Data Type Conversion2/1 -> Bus Creator/3  "StartupComp"
  Data Type Conversion1/1 -> Bus Creator/2  "DiagInput"
  Data Type Conversion/1 -> Bus Creator/1  "EnableSubsystem"
  Signal Builder/1(EnableSubsystem) -> Data Type Conversion/1
  Signal Builder/15(JumpDownEn) -> Data Type Conversion14/1
  Signal Builder/14(PreestorageFreezeTrigger) -> Data Type Conversion13/1
  Signal Builder/13(HealEnable) -> Data Type Conversion12/1
  Signal Builder/12(DiagEnable) -> Data Type Conversion11/1
  Signal Builder/11(DiagReset) -> Data Type Conversion10/1
  Signal Builder/10(DebounceEn) -> Data Type Conversion9/1
  Signal Builder/9(PassCountThd) -> Data Type Conversion8/1
  Signal Builder/8(FaultCountThd) -> Data Type Conversion7/1
  Signal Builder/7(DownCount) -> Data Type Conversion6/1
  Signal Builder/6(UpCount) -> Data Type Conversion5/1
  Signal Builder/5(MinValue) -> Data Type Conversion3/1
  Signal Builder/4(MaxValue) -> Data Type Conversion4/1
  Signal Builder/3(StartupComp) -> Data Type Conversion2/1
  Bus Creator/1 -> Out1/1
  Signal Builder/2(DiagInput) -> Data Type Conversion1/1

== system DiagCCaller_TestHarness/Debounce Enabled - RESET by Calibration ,Fault Active, FaultCnt = 10, PassCnt = 0 , Heal 0  ==
  Bus Creator : BusCreator  Inputs=15
  Data Type Conversion{,1..2,9..14} (9 alike) : DataTypeConversion  OutDataTypeStr=boolean
  Data Type Conversion3 : DataTypeConversion  OutDataTypeStr=single
  Data Type Conversion4 : DataTypeConversion  OutDataTypeStr=single
  Data Type Conversion{5..8} (4 alike) : DataTypeConversion  OutDataTypeStr=int16
  Signal Builder : Subsystem  Tag=STV Subsys  LoadFcn=sigbuilder_block('load');  StartFcn=sigbuilder_block('start');  StopFcn=sigbuilder_block('stop');  ClipboardFcn=sigbuilder_block('clipboard');  TreatAsAtomicUnit=on  mask(Sigbuilder block){tuvar=[0:10]}
      mask help: Simulink:masks:SigbuilderBlock_MD
      mask init:
      | if ~strcmp(get_param(bdroot(gcbh),'SimulationStatus'),'stopped') tuvar = sigbuilder_block('maskInit'); end
      settings: CopyFcn=sigbuilder_block('copy');  DeleteFcn=sigbuilder_block('delete');  ModelCloseFcn=sigbuilder_block('modelClose');  PreSaveFcn=sigbuilder_block('preSave');  PauseFcn=sigbuilder_block('pause');  ContinueFcn=sigbuilder_block('continue');  NameChangeFcn=sigbuilder_block('namechange');  OpenFcn=sigbuilder_block('open',[5.4 30 1141.2 522.6 ]);  CloseFcn=sigbuilder_block('close');
      mask Display: plot(0, 0, 100, 100,[2, 2, 32, 32, 2], [68, 8, 8, 68, 68],[32, 2], [38, 38], [32, 19, 2],[53, 60, 44], [32, 17, 17, 2],[16, 16, 31, 31]);txt = getActiveGroup(gcbh);text(2, 100, txt,'verticalAlignment', 'top');
  Out1 : Outport
  wires:
  Data Type Conversion14/1 -> Bus Creator/15  "JumpDownEn"
  Data Type Conversion13/1 -> Bus Creator/14  "PreestorageFreezeTrigger"
  Data Type Conversion12/1 -> Bus Creator/13  "HealEnable"
  Data Type Conversion11/1 -> Bus Creator/12  "DiagEnable"
  Data Type Conversion10/1 -> Bus Creator/11  "DiagReset"
  Data Type Conversion9/1 -> Bus Creator/10  "DebounceEn"
  Data Type Conversion8/1 -> Bus Creator/9  "PassCountThd"
  Data Type Conversion7/1 -> Bus Creator/8  "FaultCountThd"
  Data Type Conversion6/1 -> Bus Creator/7  "DownCount"
  Data Type Conversion5/1 -> Bus Creator/6  "UpCount"
  Data Type Conversion3/1 -> Bus Creator/5  "MinValue"
  Data Type Conversion4/1 -> Bus Creator/4  "MaxValue"
  Data Type Conversion2/1 -> Bus Creator/3  "StartupComp"
  Data Type Conversion1/1 -> Bus Creator/2  "DiagInput"
  Data Type Conversion/1 -> Bus Creator/1  "EnableSubsystem"
  Signal Builder/1(EnableSubsystem) -> Data Type Conversion/1
  Signal Builder/15(JumpDownEn) -> Data Type Conversion14/1
  Signal Builder/14(PreestorageFreezeTrigger) -> Data Type Conversion13/1
  Signal Builder/13(HealEnable) -> Data Type Conversion12/1
  Signal Builder/12(DiagEnable) -> Data Type Conversion11/1
  Signal Builder/11(DiagReset) -> Data Type Conversion10/1
  Signal Builder/10(DebounceEn) -> Data Type Conversion9/1
  Signal Builder/9(PassCountThd) -> Data Type Conversion8/1
  Signal Builder/8(FaultCountThd) -> Data Type Conversion7/1
  Signal Builder/7(DownCount) -> Data Type Conversion6/1
  Signal Builder/6(UpCount) -> Data Type Conversion5/1
  Signal Builder/5(MinValue) -> Data Type Conversion3/1
  Signal Builder/4(MaxValue) -> Data Type Conversion4/1
  Signal Builder/3(StartupComp) -> Data Type Conversion2/1
  Bus Creator/1 -> Out1/1
  Signal Builder/2(DiagInput) -> Data Type Conversion1/1

== system DiagCCaller_TestHarness/Debounce Enabled - RESET by Calibration ,Fault Inactive , FaultCnt = 10, PassCnt = 0 , Heal 0  ==
  Bus Creator : BusCreator  Inputs=15
  Data Type Conversion{,1..2,9..14} (9 alike) : DataTypeConversion  OutDataTypeStr=boolean
  Data Type Conversion3 : DataTypeConversion  OutDataTypeStr=single
  Data Type Conversion4 : DataTypeConversion  OutDataTypeStr=single
  Data Type Conversion{5..8} (4 alike) : DataTypeConversion  OutDataTypeStr=int16
  Signal Builder : Subsystem  Tag=STV Subsys  LoadFcn=sigbuilder_block('load');  StartFcn=sigbuilder_block('start');  StopFcn=sigbuilder_block('stop');  ClipboardFcn=sigbuilder_block('clipboard');  TreatAsAtomicUnit=on  mask(Sigbuilder block){tuvar=[0:10]}
      mask help: Simulink:masks:SigbuilderBlock_MD
      mask init:
      | if ~strcmp(get_param(bdroot(gcbh),'SimulationStatus'),'stopped') tuvar = sigbuilder_block('maskInit'); end
      settings: CopyFcn=sigbuilder_block('copy');  DeleteFcn=sigbuilder_block('delete');  ModelCloseFcn=sigbuilder_block('modelClose');  PreSaveFcn=sigbuilder_block('preSave');  PauseFcn=sigbuilder_block('pause');  ContinueFcn=sigbuilder_block('continue');  NameChangeFcn=sigbuilder_block('namechange');  OpenFcn=sigbuilder_block('open',[5.4 30 1141.2 522.6 ]);  CloseFcn=sigbuilder_block('close');
      mask Display: plot(0, 0, 100, 100,[2, 2, 32, 32, 2], [68, 8, 8, 68, 68],[32, 2], [38, 38], [32, 19, 2],[53, 60, 44], [32, 17, 17, 2],[16, 16, 31, 31]);txt = getActiveGroup(gcbh);text(2, 100, txt,'verticalAlignment', 'top');
  Out1 : Outport
  wires:
  Data Type Conversion14/1 -> Bus Creator/15  "JumpDownEn"
  Data Type Conversion13/1 -> Bus Creator/14  "PreestorageFreezeTrigger"
  Data Type Conversion12/1 -> Bus Creator/13  "HealEnable"
  Data Type Conversion11/1 -> Bus Creator/12  "DiagEnable"
  Data Type Conversion10/1 -> Bus Creator/11  "DiagReset"
  Data Type Conversion9/1 -> Bus Creator/10  "DebounceEn"
  Data Type Conversion8/1 -> Bus Creator/9  "PassCountThd"
  Data Type Conversion7/1 -> Bus Creator/8  "FaultCountThd"
  Data Type Conversion6/1 -> Bus Creator/7  "DownCount"
  Data Type Conversion5/1 -> Bus Creator/6  "UpCount"
  Data Type Conversion3/1 -> Bus Creator/5  "MinValue"
  Data Type Conversion4/1 -> Bus Creator/4  "MaxValue"
  Data Type Conversion2/1 -> Bus Creator/3  "StartupComp"
  Data Type Conversion1/1 -> Bus Creator/2  "DiagInput"
  Data Type Conversion/1 -> Bus Creator/1  "EnableSubsystem"
  Signal Builder/1(EnableSubsystem) -> Data Type Conversion/1
  Signal Builder/15(JumpDownEn) -> Data Type Conversion14/1
  Signal Builder/14(PreestorageFreezeTrigger) -> Data Type Conversion13/1
  Signal Builder/13(HealEnable) -> Data Type Conversion12/1
  Signal Builder/12(DiagEnable) -> Data Type Conversion11/1
  Signal Builder/11(DiagReset) -> Data Type Conversion10/1
  Signal Builder/10(DebounceEn) -> Data Type Conversion9/1
  Signal Builder/9(PassCountThd) -> Data Type Conversion8/1
  Signal Builder/8(FaultCountThd) -> Data Type Conversion7/1
  Signal Builder/7(DownCount) -> Data Type Conversion6/1
  Signal Builder/6(UpCount) -> Data Type Conversion5/1
  Signal Builder/5(MinValue) -> Data Type Conversion3/1
  Signal Builder/4(MaxValue) -> Data Type Conversion4/1
  Signal Builder/3(StartupComp) -> Data Type Conversion2/1
  Signal Builder/2(DiagInput) -> Data Type Conversion1/1
  Bus Creator/1 -> Out1/1

== system DiagCCaller_TestHarness/Debounce Enabled - RESET by Calibration ,Fault Inactive,  FaultCnt = 10, PassCnt = -5 , Heal 1  ==
  Bus Creator : BusCreator  Inputs=15
  Data Type Conversion{,1..2,9..14} (9 alike) : DataTypeConversion  OutDataTypeStr=boolean
  Data Type Conversion3 : DataTypeConversion  OutDataTypeStr=single
  Data Type Conversion4 : DataTypeConversion  OutDataTypeStr=single
  Data Type Conversion{5..8} (4 alike) : DataTypeConversion  OutDataTypeStr=int16
  Signal Builder : Subsystem  Tag=STV Subsys  LoadFcn=sigbuilder_block('load');  StartFcn=sigbuilder_block('start');  StopFcn=sigbuilder_block('stop');  ClipboardFcn=sigbuilder_block('clipboard');  TreatAsAtomicUnit=on  mask(Sigbuilder block){tuvar=[0:10]}
      mask help: Simulink:masks:SigbuilderBlock_MD
      mask init:
      | if ~strcmp(get_param(bdroot(gcbh),'SimulationStatus'),'stopped') tuvar = sigbuilder_block('maskInit'); end
      settings: CopyFcn=sigbuilder_block('copy');  DeleteFcn=sigbuilder_block('delete');  ModelCloseFcn=sigbuilder_block('modelClose');  PreSaveFcn=sigbuilder_block('preSave');  PauseFcn=sigbuilder_block('pause');  ContinueFcn=sigbuilder_block('continue');  NameChangeFcn=sigbuilder_block('namechange');  OpenFcn=sigbuilder_block('open',[5.4 30 1141.2 522.6 ]);  CloseFcn=sigbuilder_block('close');
      mask Display: plot(0, 0, 100, 100,[2, 2, 32, 32, 2], [68, 8, 8, 68, 68],[32, 2], [38, 38], [32, 19, 2],[53, 60, 44], [32, 17, 17, 2],[16, 16, 31, 31]);txt = getActiveGroup(gcbh);text(2, 100, txt,'verticalAlignment', 'top');
  Out1 : Outport
  wires:
  Bus Creator/1 -> Out1/1
  Signal Builder/2(DiagInput) -> Data Type Conversion1/1
  Signal Builder/3(StartupComp) -> Data Type Conversion2/1
  Signal Builder/4(MaxValue) -> Data Type Conversion4/1
  Signal Builder/5(MinValue) -> Data Type Conversion3/1
  Signal Builder/6(UpCount) -> Data Type Conversion5/1
  Signal Builder/7(DownCount) -> Data Type Conversion6/1
  Signal Builder/8(FaultCountThd) -> Data Type Conversion7/1
  Signal Builder/9(PassCountThd) -> Data Type Conversion8/1
  Signal Builder/10(DebounceEn) -> Data Type Conversion9/1
  Signal Builder/11(DiagReset) -> Data Type Conversion10/1
  Signal Builder/12(DiagEnable) -> Data Type Conversion11/1
  Signal Builder/13(HealEnable) -> Data Type Conversion12/1
  Signal Builder/14(PreestorageFreezeTrigger) -> Data Type Conversion13/1
  Signal Builder/15(JumpDownEn) -> Data Type Conversion14/1
  Signal Builder/1(EnableSubsystem) -> Data Type Conversion/1
  Data Type Conversion/1 -> Bus Creator/1  "EnableSubsystem"
  Data Type Conversion1/1 -> Bus Creator/2  "DiagInput"
  Data Type Conversion2/1 -> Bus Creator/3  "StartupComp"
  Data Type Conversion4/1 -> Bus Creator/4  "MaxValue"
  Data Type Conversion3/1 -> Bus Creator/5  "MinValue"
  Data Type Conversion5/1 -> Bus Creator/6  "UpCount"
  Data Type Conversion6/1 -> Bus Creator/7  "DownCount"
  Data Type Conversion7/1 -> Bus Creator/8  "FaultCountThd"
  Data Type Conversion8/1 -> Bus Creator/9  "PassCountThd"
  Data Type Conversion9/1 -> Bus Creator/10  "DebounceEn"
  Data Type Conversion10/1 -> Bus Creator/11  "DiagReset"
  Data Type Conversion11/1 -> Bus Creator/12  "DiagEnable"
  Data Type Conversion12/1 -> Bus Creator/13  "HealEnable"
  Data Type Conversion13/1 -> Bus Creator/14  "PreestorageFreezeTrigger"
  Data Type Conversion14/1 -> Bus Creator/15  "JumpDownEn"
